simulink model "AMCLIB_TrackObsrv_BAM"  (Simulink 9.3)
settings: Solver=VariableStepAuto  StartTime=0.0  StopTime=10.0  RelTol=1e-3
settings Model: Creator=nxa18952  LastModifiedBy=nxa18952
settings DataIOCC: SaveFormat=Dataset  SignalLoggingSaveFormat=Dataset  ReturnWorkspaceOutputs=on
settings OptimizationCC: LifeSpan=auto
settings DebuggingCC: UnderspecifiedInitializationDetection=Simplified  MergeDetectMultiDrivingBlocksExec=error  FcnCallInpInsideContextMsg=error  SFUnexpectedBacktrackingDiag=error  SFNoUnconditionalDefaultTransitionDiag=error  SFExecutionAtInitializationDiag=warning  ArithmeticOperatorsInVariantConditions=error
settings HardwareCC: ProdBitPerPointer=64  ProdBitPerSizeT=64  ProdBitPerPtrDiffT=64  ProdLargestAtomicFloat=Float  ProdIntDivRoundTo=Zero  ProdEndianess=LittleEndian  ProdWordSize=64  ProdHWDeviceType=Intel->x86-64 (Windows64)
settings ModelReferenceCC: PropagateSignalLabelsOutOfModel=on
settings SFSimCC: SimUseLocalCustomCode=on
settings RTWCC: RTWUseLocalCustomCode=on
settings CodeAppCC: StateflowObjectComments=off
settings GRTTargetCC: TargetLangStandard=C99 (ISO)  CombineOutputUpdateFcns=on  GRTInterface=off
settings ConfigComp: CovMetricSettings=dwe  CovHtmlReporting=off  CovSaveCumulativeToWorkspaceVar=off  CovSaveSingleToWorkspaceVar=off  CovExternalEMLEnable=on

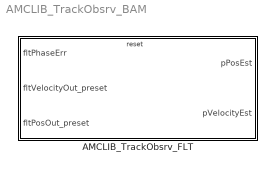
== system AMCLIB_TrackObsrv_BAM ==
  AMCLIB_TrackObsrv_FLT : Subsystem  TreatAsAtomicUnit=on  mask(AMCLIB_TrackObsrv_FLT){showStates=Hide (faster execution), resetStatesEnable=Pre-set according to the first set of inputs after reset, fltCC1sc=0, fltCC2sc=0, fltUpperLimit=0, fltLowerLimit=0, fltC1=0}
      mask prompts: showStates "Show internal states"; resetStatesEnable "Internal state after reset"; fltCC1sc "fltCC1sc (GFLIB_ControllerPIrAW - CC1 coefficient)"; fltCC2sc "fltCC2sc (GFLIB_ControllerPIrAW - CC2 coefficient)"; fltUpperLimit "fltUpperLimit (GFLIB_ControllerPIrAW - upper Limit of the controller)"; fltLowerLimit "fltLowerLimit (GFLIB_ControllerPIrAW - lower Limit of the controller)"; fltC1 "fltC1 (GFLIB_IntegratorTR - integrator coefficient)"
      mask help: Tracking observer in single precision floating-point implementation. This block supports re-initialization of the internal state during simulation. If the block is reset, the outputs of the PI controller and integrator will be aligned with the inputs fltVelocityOut_preset and fltPosOut_preset. Refer to the AMMCLIB User's Guide for further details.
      mask init:
      | if ~evalin('base','exist(''tS8'',''var'')')
      |   if (2 ~= exist('SWLIBS_Typedefs.mat','file'))
      |       error('File SWLIBS_Typedefs.mat is not on the Matlab path. Please add the AMMCLIB "bam" folder in the Matlab Search Path.');
      |   else
      |       evalin('base', 'load(''SWLIBS_Typedefs.mat'')');
      |   end
      | end
      | if showStates == 1
      |     % hidden state variables
      |     if strcmp(get_param([gcb '/fltCC1'], 'BlockType'), 'Inport')
      |         posblk = get_param(gcb, 'Position');
      | 
      |         pos = get_param(    [gcb, '/fltCC1'], 'Position');
      |         orient = get_param( [gcb, '/fltCC1'], 'Orientation');
      |         delete_block(       [gcb, '/fltCC1']);
      |         add_block('built-in/Ground', [gcb, '/fltCC1'], 'Position', pos, 'Orientation', orient);
      | 
      |         pos = get_param(    [gcb, '/fltCC2'], 'Position');
      |         orient = get_param( [gcb, '/fltCC2'], 'Orientation');
      |         delete_block(       [gcb, '/fltCC2']);
      |         add_block('built-in/Ground', [gcb, '/fltCC2'], 'Position', pos, 'Orientation', orient);
      | 
      |         pos = get_param(    [gcb, '/fltUpperLimit'], 'Position');
      |         orient = get_param( [gcb, '/fltUpperLimit'], 'Orientation');
      |         delete_block(       [gcb, '/fltUpperLimit']);
      |         add_block('built-in/Ground', [gcb, '/fltUpperLimit'], 'Position', pos, 'Orientation', orient);
      | 
      |         pos = get_param(    [gcb, '/fltLowerLimit'], 'Position');
      |         orient = get_param( [gcb, '/fltLowerLimit'], 'Orientation');
      |         delete_block(       [gcb, '/fltLowerLimit']);
      |         add_block('built-in/Ground', [gcb, '/fltLowerLimit'], 'Position', pos, 'Orientation', orient);
      | 
      |         pos = get_param(    [gcb, '/fltC1'], 'Position');
      |         orient = get_param( [gcb, '/fltC1'], 'Orientation');
      |         delete_block(       [gcb, '/fltC1']);
      |         add_block('built-in/Ground', [gcb, '/fltC1'], 'Position', pos, 'Orientation', orient);
      | 
      |         pos = get_param(    [gcb, '/fltAcc'], 'Position');
      |         orient = get_param( [gcb, '/fltAcc'], 'Orientation');
      |         delete_block(       [gcb, '/fltAcc']);
      |         add_block('built-in/Ground', [gcb, '/fltAcc'], 'Position', pos, 'Orientation', orient);
      | 
      |         pos = get_param(    [gcb, '/fltInErrK1'], 'Position');
      |         orient = get_param( [gcb, '/fltInErrK1'], 'Orientation');
      |         delete_block(       [gcb, '/fltInErrK1']);
      |         add_block('built-in/Ground', [gcb, '/fltInErrK1'], 'Position', pos, 'Orientation', orient);
      | 
      |         pos = get_param(    [gcb, '/fltState'], 'Position');
      |         orient = get_param( [gcb, '/fltState'], 'Orientation');
      |         delete_block(       [gcb, '/fltState']);
      |         add_block('built-in/Ground', [gcb, '/fltState'], 'Position', pos, 'Orientation', orient);
      | 
      |         pos = get_param(    [gcb, '/fltInK1'], 'Position');
      |         orient = get_param( [gcb, '/fltInK1'], 'Orientation');
      |         delete_block(       [gcb, '/fltInK1']);
      |         add_block('built-in/Ground', [gcb, '/fltInK1'], 'Position', pos, 'Orientation', orient);
      | 
      | 
      |         pos = get_param(    [gcb '/fltAcc_Out'], 'Position');
      |         orient = get_param( [gcb '/fltAcc_Out'], 'Orientation');
      |         delete_block(       [gcb '/fltAcc_Out']);
      |         add_block('built-in/Terminator', [gcb '/fltAcc_Out'], 'Position', pos, 'Orientation', orient);
      | 
      |         pos = get_param(    [gcb '/fltInErrK1_Out'], 'Position');
      |         orient = get_param( [gcb '/fltInErrK1_Out'], 'Orientation');
      |         delete_block(       [gcb '/fltInErrK1_Out']);
      |         add_block('built-in/Terminator', [gcb '/fltInErrK1_Out'], 'Position', pos, 'Orientation', orient);
      | 
      |         pos = get_param(    [gcb '/fltState_Out'], 'Position');
      |         orient = get_param( [gcb '/fltState_Out'], 'Orientation');
      |         delete_block(       [gcb '/fltState_Out']);
      |         add_block('built-in/Terminator', [gcb '/fltState_Out'], 'Position', pos, 'Orientation', orient);
      | 
      |         pos = get_param(    [gcb '/fltInK1_Out'], 'Position');
      |         orient = get_param( [gcb '/fltInK1_Out'], 'Orientation');
      |         delete_block(       [gcb '/fltInK1_Out']);
      |         add_block('built-in/Terminator', [gcb '/fltInK1_Out'], 'Position', pos, 'Orientation', orient);
      | 
      | 
      |         set_param([gcb '/fltPhaseErr'], 'Port', '1');
      |         set_param([gcb '/fltVelocityOut_preset'], 'Port', '2');
      |         set_param([gcb '/fltPosOut_preset'], 'Port', '3');
      | 
      |         set_param([gcb '/pPosEst'], 'Port', '1');
      |         set_param([gcb '/pVelocityEst'], 'Port', '2');
      | 
      |         set_param(gcb,'MaskEnables',{'on','on','on','on','on','on','on'});
      | 
      |         if (posblk(4) - posblk(2)) > 100
      |           height = 100;
      |           set_param(gcb,'Position',[posblk(1), posblk(2), posblk(3), posblk(2)+height])
      |         end
      |     end
      | else
      |     % shown state variables
      |     if strcmp(get_param([gcb '/fltCC1'], 'BlockType'), 'Ground')
      |         posblk = get_param(gcb, 'Position');
      | 
      |         pos = get_param(    [gcb, '/fltCC1'], 'Position');
      |         orient = get_param( [gcb, '/fltCC1'], 'Orientation');
      |         delete_block(       [gcb, '/fltCC1']);
      |         add_block('built-in/Inport', [gcb, '/fltCC1'], 'Position', pos, 'Orientation', orient, 'OutDataTypeStr', 'single');
      | 
      |         pos = get_param(    [gcb, '/fltCC2'], 'Position');
      |         orient = get_param( [gcb, '/fltCC2'], 'Orientation');
      |         delete_block(       [gcb, '/fltCC2']);
      |         add_block('built-in/Inport', [gcb, '/fltCC2'], 'Position', pos, 'Orientation', orient, 'OutDataTypeStr', 'single');
      | 
      |         pos = get_param(    [gcb, '/fltUpperLimit'], 'Position');
      |         orient = get_param( [gcb, '/fltUpperLimit'], 'Orientation');
      |         delete_block(       [gcb, '/fltUpperLimit']);
      |         add_block('built-in/Inport', [gcb, '/fltUpperLimit'], 'Position', pos, 'Orientation', orient, 'OutDataTypeStr', 'single');
      | 
      |         pos = get_param(    [gcb, '/fltLowerLimit'], 'Position');
      |         orient = get_param( [gcb, '/fltLowerLimit'], 'Orientation');
      |         delete_block(       [gcb, '/fltLowerLimit']);
      |         add_block('built-in/Inport', [gcb, '/fltLowerLimit'], 'Position', pos, 'Orientation', orient, 'OutDataTypeStr', 'single');
      | 
      |         pos = get_param(    [gcb, '/fltC1'], 'Position');
      |         orient = get_param( [gcb, '/fltC1'], 'Orientation');
      |         delete_block(       [gcb, '/fltC1']);
      |         add_block('built-in/Inport', [gcb, '/fltC1'], 'Position', pos, 'Orientation', orient, 'OutDataTypeStr', 'single');
      | 
      |         pos = get_param(    [gcb, '/fltAcc'], 'Position');
      |         orient = get_param( [gcb, '/fltAcc'], 'Orientation');
      |         delete_block(       [gcb, '/fltAcc']);
      |         add_block('built-in/Inport', [gcb, '/fltAcc'], 'Position', pos, 'Orientation', orient, 'OutDataTypeStr', 'single');
      | 
      |         pos = get_param(    [gcb, '/fltInErrK1'], 'Position');
      |         orient = get_param( [gcb, '/fltInErrK1'], 'Orientation');
      |         delete_block(       [gcb, '/fltInErrK1']);
      |         add_block('built-in/Inport', [gcb, '/fltInErrK1'], 'Position', pos, 'Orientation', orient, 'OutDataTypeStr', 'single');
      | 
      |         pos = get_param(    [gcb, '/fltState'], 'Position');
      |         orient = get_param( [gcb, '/fltState'], 'Orientation');
      |         delete_block(       [gcb, '/fltState']);
      |         add_block('built-in/Inport', [gcb, '/fltState'], 'Position', pos, 'Orientation', orient, 'OutDataTypeStr', 'single');
      | 
      |         pos = get_param(    [gcb, '/fltInK1'], 'Position');
      |         orient = get_param( [gcb, '/fltInK1'], 'Orientation');
      |         delete_block(       [gcb, '/fltInK1']);
      |         add_block('built-in/Inport', [gcb, '/fltInK1'], 'Position', pos, 'Orientation', orient, 'OutDataTypeStr', 'single');
      | 
      | 
      |         pos = get_param(    [gcb '/fltAcc_Out'], 'Position');
      |         orient = get_param( [gcb '/fltAcc_Out'], 'Orientation');
      |         delete_block(       [gcb '/fltAcc_Out']);
      |         add_block('built-in/Outport', [gcb '/fltAcc_Out'], 'Position', pos, 'Orientation', orient);
      | 
      |         pos = get_param(    [gcb '/fltInErrK1_Out'], 'Position');
      |         orient = get_param( [gcb '/fltInErrK1_Out'], 'Orientation');
      |         delete_block(       [gcb '/fltInErrK1_Out']);
      |         add_block('built-in/Outport', [gcb '/fltInErrK1_Out'], 'Position', pos, 'Orientation', orient);
      | 
      |         pos = get_param(    [gcb '/fltState_Out'], 'Position');
      |         orient = get_param( [gcb '/fltState_Out'], 'Orientation');
      |         delete_block(       [gcb '/fltState_Out']);
      |         add_block('built-in/Outport', [gcb '/fltState_Out'], 'Position', pos, 'Orientation', orient);
      | 
      |         pos = get_param(    [gcb '/fltInK1_Out'], 'Position');
      |         orient = get_param( [gcb '/fltInK1_Out'], 'Orientation');
      |         delete_block(       [gcb '/fltInK1_Out']);
      |         add_block('built-in/Outport', [gcb '/fltInK1_Out'], 'Position', pos, 'Orientation', orient);
      | 
      | 
      |         set_param([gcb '/fltPhaseErr'], 'Port', '1');
      |         set_param([gcb '/fltVelocityOut_preset'], 'Port', '2');
      |         set_param([gcb '/fltPosOut_preset'], 'Port', '3');
      |         set_param([gcb '/fltCC1'], 'Port', '4');
      |         set_param([gcb '/fltCC2'], 'Port', '5');
      |         set_param([gcb '/fltUpperLimit'], 'Port', '6');
      |         set_param([gcb '/fltLowerLimit'], 'Port', '7');
      |         set_param([gcb '/fltC1'], 'Port', '8');
      |         set_param([gcb '/fltAcc'], 'Port', '9');
      |         set_param([gcb '/fltInErrK1'], 'Port', '10');
      |         set_param([gcb '/fltState'], 'Port', '11');
      |         set_param([gcb '/fltInK1'], 'Port', '12');
      | 
      |         set_param([gcb '/pPosEst'], 'Port', '1');
      |         set_param([gcb '/pVelocityEst'], 'Port', '2');
      |         set_param([gcb '/fltAcc_Out'], 'Port', '3');
      |         set_param([gcb '/fltInErrK1_Out'], 'Port', '4');
      |         set_param([gcb '/fltState_Out'], 'Port', '5');
      |         set_param([gcb '/fltInK1_Out'], 'Port', '6');
      | 
      |         set_param(gcb,'MaskEnables',{'on','on','off','off','off','off','off'});
      | 
      |         if (posblk(4) - posblk(2)) < 325
      |           height = 325;
      |           set_param(gcb,'Position',[posblk(1), posblk(2), posblk(3), posblk(2)+height])
      |         end
      |     end
      | end
      settings: RTWSystemCode=Inline
      mask TypeOptions showStates: Hide (faster execution) | Show (allows debugging; connect feedback loops manually)
      mask Callback showStates:
      | maskStr = get_param(gcb,'showStates');
      | if strcmp(maskStr,'Hide (faster execution)'),
      |     set_param(gcb,'MaskEnables',{'on','on','on','on','on','on','on'});
      | else
      |     set_param(gcb,'MaskEnables',{'on','on','off','off','off','off','off'});
      | end
      mask TypeOptions resetStatesEnable: Pre-set according to the first set of inputs after reset | Clear to zero
      mask Display:
      | color('black');
      | pos = get_param(gcb, 'Position');
      | width = pos(3) - pos(1);
      | height = pos(4) - pos(2);
      | tX=width/2;
      | tY=height - 25;
      | color('black');
      | text(tX,tY, 'AMCLIB_TrackObsrv_FLT', 'horizontalAlignment', 'center');
      | if showStates == 2
      |   color('red');
      |   text(tX,tY - 20, ['debugging mode' char(13) char(10) '(limited performance)'], 'horizontalAlignment', 'center');
      | end

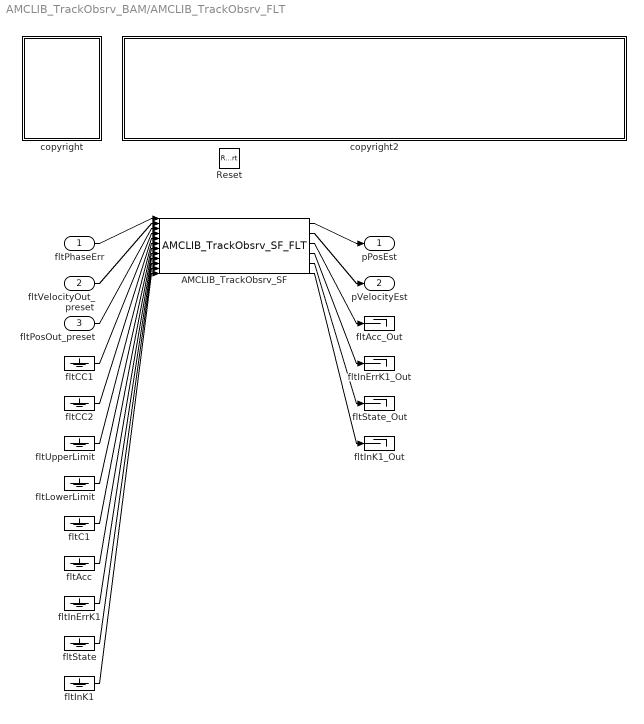
== system AMCLIB_TrackObsrv_BAM/AMCLIB_TrackObsrv_FLT ==
  fltPhaseErr : Inport  OutDataTypeStr=single
  fltVelocityOut_preset : Inport  Port=2  OutDataTypeStr=single
  fltPosOut_preset : Inport  Port=3  OutDataTypeStr=single
  Reset : ResetPort  DisableCoverage=on
  AMCLIB_TrackObsrv_SF : S-Function  FunctionName=AMCLIB_TrackObsrv_SF_FLT  Parameters=showStates,resetStatesEnable,fltCC1sc,fltCC2sc,fltUpperLimit,fltLowerLimit,fltC1  SFunctionDeploymentMode=off  EnableBusSupport=off
  copyright : Subsystem
      mask Display: text(10,90,'FILE:');text(10,75,'DESRIPTION:');text(10,60,'COPYRIGHT:');text(10,45,'VERSION:');text(10,30,'DATE:')
  copyright2 : Subsystem
      mask Display: text(10,90,'AMCLIB_TrackObsrv_BAM_FLT.mdl');text(10,75,'Tracking observer');text(10,60,'NXP 2020');text(10,45,'1.0');text(10,30,'28-Mar-2020');
  fltAcc : Ground
  fltAcc_Out : Terminator
  fltC1 : Ground
  fltCC1 : Ground
  fltCC2 : Ground
  fltInErrK1 : Ground
  fltInErrK1_Out : Terminator
  fltInK1 : Ground
  fltInK1_Out : Terminator
  fltLowerLimit : Ground
  fltState : Ground
  fltState_Out : Terminator
  fltUpperLimit : Ground
  pPosEst : Outport
  pVelocityEst : Outport  Port=2
  wires:
  fltPhaseErr/1 -> AMCLIB_TrackObsrv_SF/1
  fltVelocityOut_preset/1 -> AMCLIB_TrackObsrv_SF/2
  fltPosOut_preset/1 -> AMCLIB_TrackObsrv_SF/3
  fltCC1/1 -> AMCLIB_TrackObsrv_SF/4
  fltCC2/1 -> AMCLIB_TrackObsrv_SF/5
  fltUpperLimit/1 -> AMCLIB_TrackObsrv_SF/6
  fltLowerLimit/1 -> AMCLIB_TrackObsrv_SF/7
  fltC1/1 -> AMCLIB_TrackObsrv_SF/8
  fltAcc/1 -> AMCLIB_TrackObsrv_SF/9
  fltInErrK1/1 -> AMCLIB_TrackObsrv_SF/10
  fltState/1 -> AMCLIB_TrackObsrv_SF/11
  fltInK1/1 -> AMCLIB_TrackObsrv_SF/12
  AMCLIB_TrackObsrv_SF/1 -> pPosEst/1
  AMCLIB_TrackObsrv_SF/2 -> pVelocityEst/1
  AMCLIB_TrackObsrv_SF/3 -> fltAcc_Out/1
  AMCLIB_TrackObsrv_SF/4 -> fltInErrK1_Out/1
  AMCLIB_TrackObsrv_SF/5 -> fltState_Out/1
  AMCLIB_TrackObsrv_SF/6 -> fltInK1_Out/1

== system AMCLIB_TrackObsrv_BAM/AMCLIB_TrackObsrv_FLT/copyright ==

== system AMCLIB_TrackObsrv_BAM/AMCLIB_TrackObsrv_FLT/copyright2 ==
